simulink model "counter_3"  (R2019a)
settings: Solver=FixedStepDiscrete  StartTime=0.0  StopTime=50  FixedStep=1  RelTol=1e-3
settings Model: Creator=Admin  LastModifiedBy=Admin

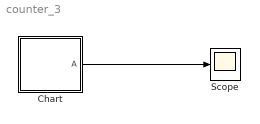
== system counter_3 ==
  Chart : Stateflow chart  BlockKeywords=__PRM__SERIALIZED__DATA__:Stateflow Chart,Stateflow Diagram  TreatAsAtomicUnit=on
  Scope : Scope
  wires:
  Chart/1(A) -> Scope/1

== stateflow chart counter_3/Chart ==
  state counter
    en :A=0;
    du: A=A+1;
  state counter_2
    en: A=-5;
    du: A=A+1;
  (default) -> counter
  counter -> counter_2 : [A==5]
  counter_2 -> counter_2 : [A==5]
  data: A output
